simulink model "LQR_try"  (R2024b)
settings: Solver=VariableStepAuto  StartTime=0.0  StopTime=10.0  RelTol=1e-3
undefined symbols (not defined in the file): gaussian
libraries: simulink x1
settings Model: Creator=SURYA  LastModifiedBy=SURYA

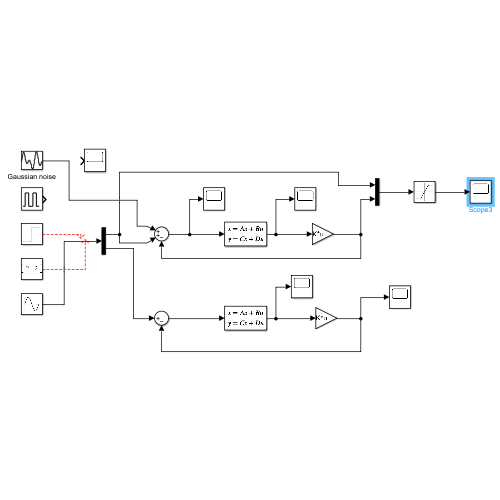
[thumbnail: Simulink's stored preview of the top-level diagram]
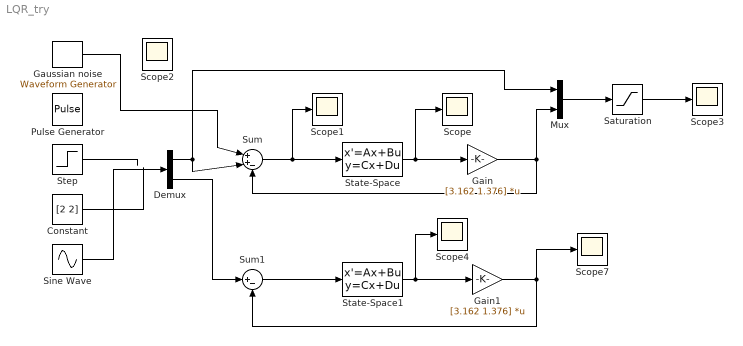
== system LQR_try ==
  Constant : Constant  Value=[2 2]
  Demux : Demux  Outputs=2
  Gain : Gain  Gain=[3.162 1.376]  Multiplication=Matrix(K*u)
  Gain1 : Gain  Gain=[3.162 1.376]  Multiplication=Matrix(K*u)
  Gaussian noise : simulink/Sources/Waveform Generator  OutMin=[]  OutMax=[]  OutDataTypeStr=double  SelectedSignal=1  Signals=gaussian('Mean', 0, 'Variance', 0.0001, 'Seed', 0)  BlockNames=MultiportSwitch_04da44c66e3142f  SampleTime=0.1
  Mux : Mux  Inputs=2
  Pulse Generator : DiscretePulseGenerator  PulseType=Time based  Amplitude=[1 1]  Period=10  PulseWidth=5
  Saturation : Saturate  UpperLimit=6
  Scope{,1..4,7} (6 alike) : Scope
  Sine Wave : Sin  Amplitude=[1 1]  SampleTime=0
  State-Space : StateSpace  A=[0 1; 0 0]  B=[0; 7.07]  C=[1 0; 0 1]  D=[0; 0]  InitialCondition=[0; 0]
  State-Space1 : StateSpace  A=[0 1; 0 0]  B=[0; 7.07]  C=[1 0; 0 1]  D=[0; 0]  InitialCondition=[0; 0]
  Step : Step  Before=[0 0]  After=[1 1]  SampleTime=0
  Sum : Sum  Inputs=|++-
  Sum1 : Sum  Inputs=|+-
  wires:
  Sum/1 -> Scope1/1, State-Space/1
  State-Space/1 -> Scope/1, Gain/1
  Demux/1 -> Mux/1, Sum/2
  Gain/1 -> Mux/2, Sum/3
  State-Space1/1 -> Gain1/1, Scope4/1
  Sum1/1 -> State-Space1/1
  Demux/2 -> Sum1/1
  Gain1/1 -> Sum1/2, Scope7/1
  Step/1 -> ?
  Mux/1 -> Saturation/1
  Saturation/1 -> Scope3/1
  Constant/1 -> ?
  Gaussian noise/1 -> Sum/1
  Sine Wave/1 -> Demux/1
